simulink library "forceslib"  (R2020b)
settings: Solver=VariableStepAuto  StartTime=0.0  StopTime=10.0  RelTol=1e-3
undefined symbols (not defined in the file or in its folder): forcesnlmpcblock_InitFcn
settings Model: Creator=rchen  LastModifiedBy=NivethanYogarajah

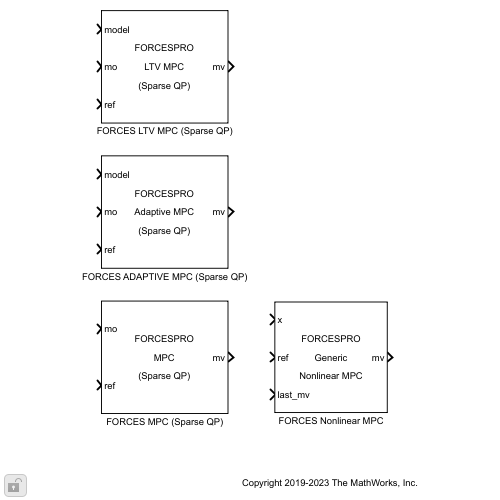
[thumbnail: Simulink's stored preview of the top-level diagram]
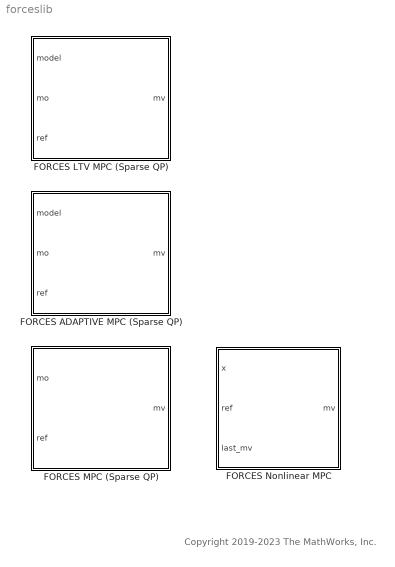
== system forceslib ==
  note: Copyright 2019-2023 The MathWorks, Inc.
  FORCES ADAPTIVE MPC (Sparse QP) : Subsystem  InitFcn=forcesmpcblock_InitFcn  mask(ForcesAdaptiveMPC_SparseQP){CoreData=[], StateData=[], md_inport=off, mv_inport=off, uref_inport=off, state_inport=off, ymin_inport=off, ymax_inport=off, umin_inport=off, umax_inport=off, dumin_inport=off, dumax_inport=off, ywt_inport=off, uwt_inport=off, duwt_inport=off, ecrwt_inport=off, return_cost=off, return_mvseq=off, return_qpstatus=off, return_qpsolvetime=off, return_solverid=off, return_xseq=off, return_state=off, return_yseq=off}
      mask prompts: CoreData "Core Data"; StateData "Initial State Data"; md_inport "Measured disturbance (md)"; mv_inport "External manipulated variable (ext.mv)"; uref_inport "References for manipulated variables (mv.target)"; state_inport "Use custom state estimation (x[k|k])"; ymin_inport "Lower OV Limits (ymin)"; ymax_inport "Upper OV Limits (ymax)"; umin_inport "Lower MV Limits (umin)"; umax_inport "Upper MV Limits (umax)"; dumin_inport "Lower MVRate Limits (dumin)"; dumax_inport "Upper MVRate Limits (dumax)"; ywt_inport "OV Weights (y.wt)"; uwt_inport "MV Weights (u.wt)"; duwt_inport "MVRate Weights (du.wt)"; ecrwt_inport "Slack Variable Weight (ecr.wt)"; return_cost "Optimal cost (cost)"; return_mvseq "Optimal control sequence (mv.seq)"; return_qpstatus "Optimization status (qp.status)"; return_qpsolvetime "Optimization solvetime (qp.solvetime)"; return_solverid "Solver Id (solverid)"; return_xseq "Optimal state sequence (x.seq)"; return_state "Estimated current states (est.state)"; return_yseq "Optimal output sequence (y.seq)"
      mask help:
      | Simulate adaptive MPC controller and generate code  using FORCESPRO QP solver.
      |
      | In MATLAB, use the following commands to generate custom FORCES QP solver from your MPC controller (mpcobj):
      |     options = mpcToForcesOptions('sparse');
      |     options.UseAdaptive = 1;
      |     [coredata, statedata, onlinedata] = mpcToForces(mpcobj, options);
      | You can enable additional online features via the "options".
      |
      | Afterwards, specify "coredata" and "statedata" in the block dialog and enable additional input and output signals in the block that must be consistent with "options".
      mask init:
      | BlockDataType = 'double';
      | MPCstruct = forcesmpcblock_MaskInitFcn(gcb);
      mask DialogControl Container5 Prompt: Additional Signal Configuration
      mask DialogControl Container7 Prompt: State Estimation
      mask DialogControl Container3 Prompt: Online Constraints
      mask DialogControl Container4 Prompt: Online Weights
      mask DialogControl Container9 Prompt: Additional Output Signals
      mask Display:
      | fprintf('FORCESPRO\n\nAdaptive MPC\n\n(Sparse QP)');
      | port_label('output', 1, 'mv')
      | port_label('input', 1, 'model')
      | port_label('input', 2, 'mo')
      | port_label('input', 3, 'ref')
  FORCES LTV MPC (Sparse QP) : Subsystem  InitFcn=forcesmpcblock_InitFcn  mask(ForcesLTVMPC_SparseQP){CoreData=[], StateData=[], md_inport=off, mv_inport=off, uref_inport=off, state_inport=off, ymin_inport=off, ymax_inport=off, umin_inport=off, umax_inport=off, dumin_inport=off, dumax_inport=off, ywt_inport=off, uwt_inport=off, duwt_inport=off, ecrwt_inport=off, return_cost=off, return_mvseq=off, return_qpstatus=off, return_qpsolvetime=off, return_solverid=off, return_xseq=off, return_state=off, return_yseq=off}
      mask prompts: CoreData "Core Data"; StateData "Initial State Data"; md_inport "Measured disturbance (md)"; mv_inport "External manipulated variable (ext.mv)"; uref_inport "References for manipulated variables (mv.target)"; state_inport "Use custom state estimation (x[k|k])"; ymin_inport "Lower OV Limits (ymin)"; ymax_inport "Upper OV Limits (ymax)"; umin_inport "Lower MV Limits (umin)"; umax_inport "Upper MV Limits (umax)"; dumin_inport "Lower MVRate Limits (dumin)"; dumax_inport "Upper MVRate Limits (dumax)"; ywt_inport "OV Weights (y.wt)"; uwt_inport "MV Weights (u.wt)"; duwt_inport "MVRate Weights (du.wt)"; ecrwt_inport "Slack Variable Weight (ecr.wt)"; return_cost "Optimal cost (cost)"; return_mvseq "Optimal control sequence (mv.seq)"; return_qpstatus "Optimization status (qp.status)"; return_qpsolvetime "Optimization solvetime (qp.solvetime)"; return_solverid "Solver Id (solverid)"; return_xseq "Optimal state sequence (x.seq)"; return_state "Estimated current states (est.state)"; return_yseq "Optimal output sequence (y.seq)"
      mask help:
      | Simulate time-varying MPC controller and generate code  using FORCESPRO QP solver.
      |
      | In MATLAB, use the following commands to generate custom FORCES QP solver from your MPC controller (mpcobj):
      |     options = mpcToForcesOptions('sparse');
      |     options.UseLTV = 1;
      |     [coredata, statedata, onlinedata] = mpcToForces(mpcobj, options);
      | You can enable additional online features via the "options".
      |
      | Afterwards, specify "coredata" and "statedata" in the block dialog and enable additional input and output signals in the block that must be consistent with "options".
      mask init:
      | BlockDataType = 'double';
      | MPCstruct = forcesmpcblock_MaskInitFcn(gcb);
      mask DialogControl Container5 Prompt: Additional Signal Configuration
      mask DialogControl Container7 Prompt: State Estimation
      mask DialogControl Container3 Prompt: Online Constraints
      mask DialogControl Container4 Prompt: Online Weights
      mask DialogControl Container9 Prompt: Additional Output Signals
      mask Display:
      | fprintf('FORCESPRO\n\nLTV MPC\n\n(Sparse QP)');
      | port_label('output', 1, 'mv')
      | port_label('input', 1, 'model')
      | port_label('input', 2, 'mo')
      | port_label('input', 3, 'ref')
  FORCES MPC (Sparse QP) : Subsystem  InitFcn=forcesmpcblock_InitFcn  mask(ForcesMPC_SparseQP){CoreData=[], StateData=[], md_inport=off, mv_inport=off, uref_inport=off, state_inport=off, ymin_inport=off, ymax_inport=off, umin_inport=off, umax_inport=off, dumin_inport=off, dumax_inport=off, ywt_inport=off, uwt_inport=off, duwt_inport=off, ecrwt_inport=off, return_cost=off, return_mvseq=off, return_qpstatus=off, return_qpsolvetime=off, return_solverid=off, return_xseq=off, return_state=off, return_yseq=off}
      mask prompts: CoreData "Core Data"; StateData "Initial State Data"; md_inport "Measured disturbance (md)"; mv_inport "External manipulated variable (ext.mv)"; uref_inport "References for manipulated variables (mv.target)"; state_inport "Use custom state estimation (x[k|k])"; ymin_inport "Lower OV Limits (ymin)"; ymax_inport "Upper OV Limits (ymax)"; umin_inport "Lower MV Limits (umin)"; umax_inport "Upper MV Limits (umax)"; dumin_inport "Lower MVRate Limits (dumin)"; dumax_inport "Upper MVRate Limits (dumax)"; ywt_inport "OV Weights (y.wt)"; uwt_inport "MV Weights (u.wt)"; duwt_inport "MVRate Weights (du.wt)"; ecrwt_inport "Slack Variable Weight (ecr.wt)"; return_cost "Optimal cost (cost)"; return_mvseq "Optimal control sequence (mv.seq)"; return_qpstatus "Optimization status (qp.status)"; return_qpsolvetime "Optimization solvetime (qp.solvetime)"; return_solverid "Solver Id (solverid)"; return_xseq "Optimal state sequence (x.seq)"; return_state "Estimated current states (est.state)"; return_yseq "Optimal output sequence (y.seq)"
      mask help:
      | Simulate MPC controller and generate code  using FORCESPRO QP solver.
      |
      | In MATLAB, use the following commands to generate custom FORCES QP solver from your MPC controller (mpcobj):
      |     options = mpcToForcesOptions('sparse');
      |     [coredata, statedata, onlinedata] = mpcToForces(mpcobj, options);
      | You can enable additional online features via the "options".
      |
      | Afterwards, specify "coredata" and "statedata" in the block dialog and enable additional input and output signals in the block that must be consistent with "options".
      mask init:
      | BlockDataType = 'double';
      | MPCstruct = forcesmpcblock_MaskInitFcn(gcb);
      mask DialogControl Container5 Prompt: Additional Signal Configuration
      mask DialogControl Container7 Prompt: State Estimation
      mask DialogControl Container3 Prompt: Online Constraints
      mask DialogControl Container4 Prompt: Online Weights
      mask DialogControl Container9 Prompt: Additional Output Signals
      mask Display:
      | fprintf('FORCESPRO\n\nMPC\n\n(Sparse QP)');
      | port_label('output', 1, 'mv')
      | port_label('input', 1, 'mo')
      | port_label('input', 2, 'ref')
  FORCES Nonlinear MPC : Subsystem  SCDEnableBlockLinearizationSpecification=on  InitFcn=forcesnlmpcblock_InitFcn;  mask(NonlinearMPC_FORCESPRO){nlmpcobj=, UseObjectTs=on, TsControl=, md_enabled=off, mvtarget_enabled=off, param_enabled=off, cost_enabled=off, mvseq_enabled=off, stateseq_enabled=off, ovseq_enabled=off, status_enabled=off, solvetime_enabled=off, solverid_enabled=off, ov_min=off, ov_max=off, mv_min=off, mv_max=off, mvrate_min=off, mvrate_max=off, state_min=off, state_max=off, ov_weight=off, mv_weight=off, mvrate_weight=off, ecr_weight=off, nlp_initialize=off}
      mask prompts: nlmpcobj ""coredata" structure generated from "nlmpcToForces""; UseObjectTs "Use prediction model sample time"; TsControl "Controller sample time (can be faster than prediction model sample time)"; md_enabled "Measured disturbances (md)"; mvtarget_enabled "MV targets (mv.target)"; param_enabled "Model parameters (param)"; cost_enabled "Optimal cost (cost)"; mvseq_enabled "Optimal control sequence (mv.seq)"; stateseq_enabled "Optimal state sequence (x.seq)"; ovseq_enabled "Optimal output sequence (y.seq)"; status_enabled "Optimization status (nlp.status)"; solvetime_enabled "Optimization solvetime (nlp.solvetime)"; solverid_enabled "Solver Id (solverid)"; ov_min "Lower OV limits (y.min)"; ov_max "Upper OV limits (y.max)"; mv_min "Lower MV limits (mv.min)"; mv_max "Upper MV limits (mv.max)"; mvrate_min "Lower MVRate limits (dmv.min)"; mvrate_max "Upper MVRate limits (dmv.max)"; state_min "Lower state limits (x.min)"; state_max "Upper state limits (x.max)"; ov_weight "OV weights (y.wt)"; mv_weight "MV weights (mv.wt)"; mvrate_weight "MVRate weights (dmv.wt)"; ecr_weight "ECR weight (ecr.wt)"; nlp_initialize "Initial guess (mv.init, x.init)"
      mask help:
      | Simulate nonlinear MPC controller designed with "nlmpc" object from MathWorks MPC Toolbox and generate code using FORCESPRO NLP solver.
      |
      | In MATLAB, use the following commands to generate FORCES NLP solver from your "nlmpc" controller (nlobj):
      |     options = nlmpcToForcesOptions();
      |     coredata = nlmpcToForces(nlobj, options);
      | You can enable additional online features via the "options".
      |
      | Afterwards, specify "coredata" in the block dialog and enable additional input and output signals in the block that must be consistent with "options".
      mask init:
      | BlockDataType = 'double';
      | blkData = forcesnlmpcblock_MaskInitFcn(gcb);
      mask Callback UseObjectTs: nlmpc.callbackBlockCustomSampleTime(gcb);
      mask DialogControl nlmpcobj Tooltip: Specify the "coredata" structure available in MATLAB workspace or Model workspace.
      mask DialogControl Container23 Prompt: Controller Sample Time
      mask DialogControl UseObjectTs Tooltip: Select if you want to run the Nonlinear MPC block using the same sample time as the prediction model sample time defined in the nlmpc object (a typical situation).
      mask DialogControl TsControl Tooltip: If you want to run the Nonlinear MPC block using sample time faster than the prediction model sample time defined in the nlmpc object, specify it here.
      mask DialogControl OptionGroup Prompt: Block Options
      mask DialogControl GeneralTab Prompt: General
      mask DialogControl Container6 Prompt: Additional Inports
      mask DialogControl md_enabled Tooltip: Select if the nlmpc object has measured disturbance (MD) channels. Connect MD signals to this input port.
      mask DialogControl mvtarget_enabled Tooltip: Select if you want to specify MV references at run time. Connect a [1..p]-by-nmv signal to the input port.
      mask DialogControl param_enabled Tooltip: Select if the nlmpc object has a model parameter and connect it with a vector signal
      mask DialogControl Container7 Prompt: Additional Outports
      mask DialogControl cost_enabled Tooltip: Select if you want to access the optimal cost as a scalar signal.
      mask DialogControl mvseq_enabled Tooltip: Select if you want to access the optimal control move trajectory as a (p+1)-by-nmv signal.
      mask DialogControl stateseq_enabled Tooltip: Select if you want to access the predicted state trajectory as a (p+1)-by-nx signal.
      mask DialogControl ovseq_enabled Tooltip: Select if you want to access the predicted output trajectory as a (p+1)-by-ny signal.
      mask DialogControl status_enabled Tooltip: Select if you want to access the optimization status as a scalar signal. A positive integer indicates the solver found an optimal solution. A negative integer indicates the solver failed to find a solution, and the mv output was frozen. Zero value indicates that the maximum number of iterations was exceeded.
      mask DialogControl solvetime_enabled Tooltip: Select if you want to access the optimization status as a scalar signal. A positive integer indicates the solver found an optimal solution. A negative integer indicates the solver failed to find a solution, and the mv output was frozen. Zero value indicates that the maximum number of iterations was exceeded.
      mask DialogControl solverid_enabled Tooltip: Select if you want to access the optimization status as a scalar signal. A positive integer indicates the solver found an optimal solution. A negative integer indicates the solver failed to find a solution, and the mv output was frozen. Zero value indicates that the maximum number of iterations was exceeded.
      mask DialogControl OnlineTab Prompt: Online Features
      mask DialogControl Container6_copy Prompt: Constraints
      mask DialogControl ov_min Tooltip: Select if you want to change the minimum OV bound at run time. Connect a [1..p]-by-ny signal to the input port.
      mask DialogControl ov_max Tooltip: Select if you want to change the maximum OV bound at run time. Connect a [1..p]-by-ny signal to the input port.
      mask DialogControl mv_min Tooltip: Select if you want to change the minimum MV bound at run time. Connect a [1..p]-by-nmv signal to the input port.
      mask DialogControl mv_max Tooltip: Select if you want to change the maximum MV bound at run time. Connect a [1..p]-by-nmv signal to the input port.
      mask DialogControl mvrate_min Tooltip: Select if you want to change the minimum MVRate bound at run time. Connect a [1..p]-by-nmv signal to the input port.
      mask DialogControl mvrate_max Tooltip: Select if you want to change the maximum MVRate bound at run time. Connect a [1..p]-by-nmv signal to the input port.
      mask DialogControl state_min Tooltip: Select if you want to change the minimum state bound at run time. Connect a [1..p]-by-nx signal to the input port.
      mask DialogControl state_max Tooltip: Select if you want to change the maximum state bound at run time. Connect a [1..p]-by-nx signal to the input port.
      mask DialogControl Container7_copy Prompt: Weights
      mask DialogControl ov_weight Tooltip: Select if you want to change OV weights at run time. Connect a (1..p)-by-ny signal to the input port.
      mask DialogControl mv_weight Tooltip: Select if you want to change MV weights at run time. Connect a (1..p)-by-nmv signal to the input port.
      mask DialogControl mvrate_weight Tooltip: Select if you want to change MVRate weights at run time. Connect a (1..p)-by-nmv signal to the input port.
      mask DialogControl ecr_weight Tooltip: Select if you want to change ECR weight at run time. Connect a scalar signal to the input port.
      mask DialogControl Container13 Prompt: Others
      mask DialogControl nlp_initialize Tooltip: Select if you want to provide your own initial guess for the decision variables used in optimization at run time. Connect a "p-by-nx" signal to "x.init" and a "p-by-nmv" signal to "mv.init".
      mask Display:
      | fprintf('FORCESPRO\n\nGeneric\n\nNonlinear MPC');
      | port_label('output', 1, 'mv')
      | port_label('input', 1, 'x')
      | port_label('input', 2, 'ref')
      | port_label('input', 3, 'last_mv')

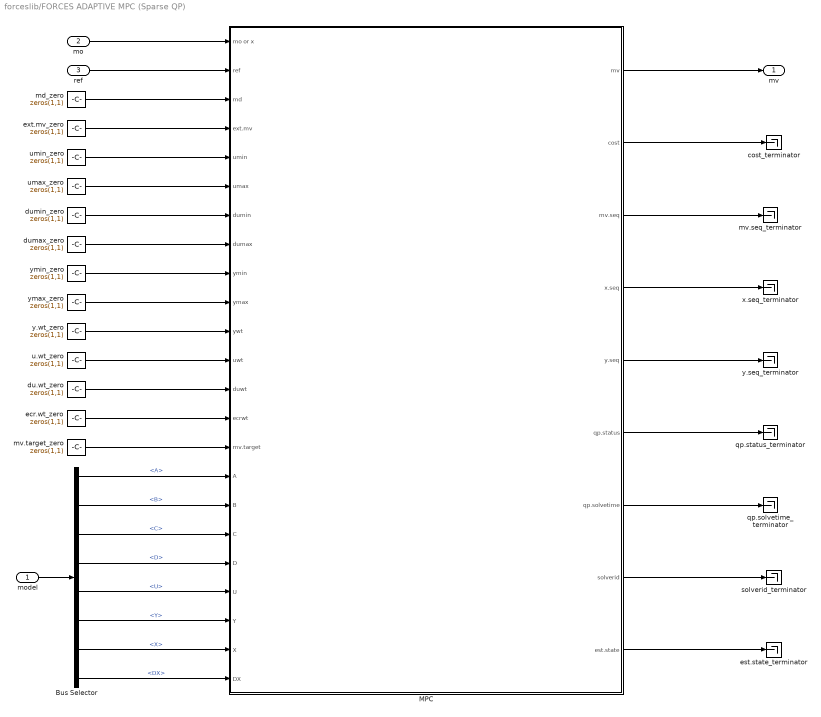
== system forceslib/FORCES ADAPTIVE MPC (Sparse QP) ==
  model : Inport
  mo : Inport  Port=2
  ref : Inport  Port=3
  Bus Selector : BusSelector  OutputSignals=A,B,C,D,U,Y,X,DX
  MPC : Subsystem
  cost_terminator : Terminator
  du.wt_zero : Constant  Value=zeros(1,1)  OutDataTypeStr=BlockDataType  SampleTime=-1
  dumax_zero : Constant  Value=zeros(1,1)  OutDataTypeStr=BlockDataType  SampleTime=-1
  dumin_zero : Constant  Value=zeros(1,1)  OutDataTypeStr=BlockDataType  SampleTime=-1
  ecr.wt_zero : Constant  Value=zeros(1,1)  OutDataTypeStr=BlockDataType  SampleTime=-1
  est.state_terminator : Terminator
  ext.mv_zero : Constant  Value=zeros(1,1)  OutDataTypeStr=BlockDataType  SampleTime=-1
  md_zero : Constant  Value=zeros(1,1)  OutDataTypeStr=BlockDataType  SampleTime=-1
  mv.seq_terminator : Terminator
  mv.target_zero : Constant  Value=zeros(1,1)  OutDataTypeStr=BlockDataType  SampleTime=-1
  qp.solvetime_terminator : Terminator
  qp.status_terminator : Terminator
  solverid_terminator : Terminator
  u.wt_zero : Constant  Value=zeros(1,1)  OutDataTypeStr=BlockDataType  SampleTime=-1
  umax_zero : Constant  Value=zeros(1,1)  OutDataTypeStr=BlockDataType  SampleTime=-1
  umin_zero : Constant  Value=zeros(1,1)  OutDataTypeStr=BlockDataType  SampleTime=-1
  x.seq_terminator : Terminator
  y.seq_terminator : Terminator
  y.wt_zero : Constant  Value=zeros(1,1)  OutDataTypeStr=BlockDataType  SampleTime=-1
  ymax_zero : Constant  Value=zeros(1,1)  OutDataTypeStr=BlockDataType  SampleTime=-1
  ymin_zero : Constant  Value=zeros(1,1)  OutDataTypeStr=BlockDataType  SampleTime=-1
  mv : Outport
  wires:
  MPC/7(qp.solvetime) -> qp.solvetime_terminator/1
  MPC/6(qp.status) -> qp.status_terminator/1
  MPC/5(y.seq) -> y.seq_terminator/1
  MPC/4(x.seq) -> x.seq_terminator/1
  MPC/3(mv.seq) -> mv.seq_terminator/1
  MPC/2(cost) -> cost_terminator/1
  mv.target_zero/1 -> MPC/15(mv.target)
  ecr.wt_zero/1 -> MPC/14(ecrwt)
  du.wt_zero/1 -> MPC/13(duwt)
  u.wt_zero/1 -> MPC/12(uwt)
  y.wt_zero/1 -> MPC/11(ywt)
  ymax_zero/1 -> MPC/10(ymax)
  ymin_zero/1 -> MPC/9(ymin)
  dumax_zero/1 -> MPC/8(dumax)
  dumin_zero/1 -> MPC/7(dumin)
  umax_zero/1 -> MPC/6(umax)
  umin_zero/1 -> MPC/5(umin)
  ext.mv_zero/1 -> MPC/4(ext.mv)
  md_zero/1 -> MPC/3(md)
  MPC/1(mv) -> mv/1
  ref/1 -> MPC/2(ref)
  mo/1 -> MPC/1(mo or x)
  MPC/9(est.state) -> est.state_terminator/1
  MPC/8(solverid) -> solverid_terminator/1
  model/1 -> Bus Selector/1
  Bus Selector/1 -> MPC/16(A)  "<A>"
  Bus Selector/2 -> MPC/17(B)  "<B>"
  Bus Selector/3 -> MPC/18(C)  "<C>"
  Bus Selector/4 -> MPC/19(D)  "<D>"
  Bus Selector/5 -> MPC/20(U)  "<U>"
  Bus Selector/6 -> MPC/21(Y)  "<Y>"
  Bus Selector/7 -> MPC/22(X)  "<X>"
  Bus Selector/8 -> MPC/23(DX)  "<DX>"

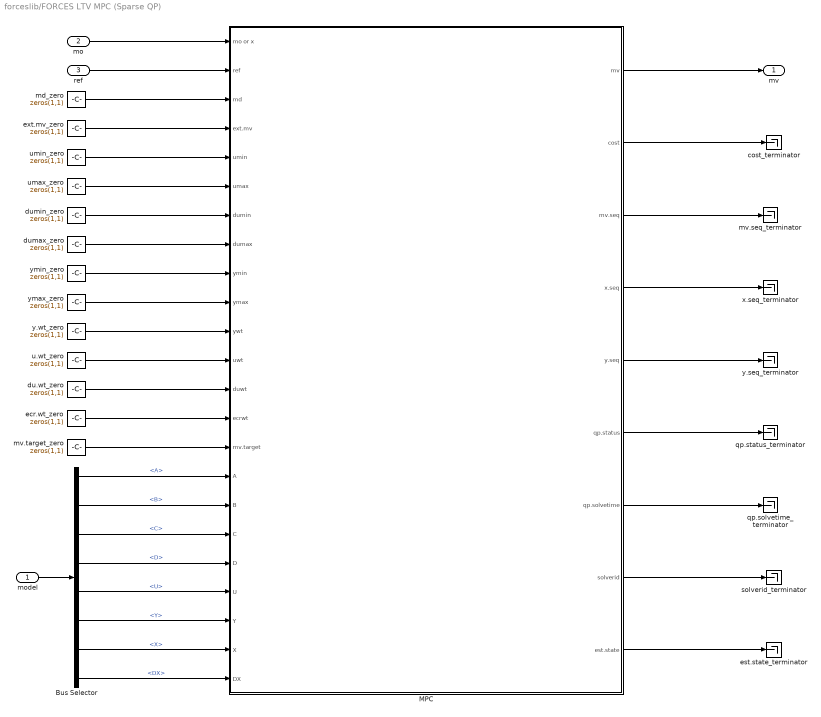
== system forceslib/FORCES LTV MPC (Sparse QP) ==
  model : Inport
  mo : Inport  Port=2
  ref : Inport  Port=3
  Bus Selector : BusSelector  OutputSignals=A,B,C,D,U,Y,X,DX
  MPC : Subsystem
  cost_terminator : Terminator
  du.wt_zero : Constant  Value=zeros(1,1)  OutDataTypeStr=BlockDataType  SampleTime=-1
  dumax_zero : Constant  Value=zeros(1,1)  OutDataTypeStr=BlockDataType  SampleTime=-1
  dumin_zero : Constant  Value=zeros(1,1)  OutDataTypeStr=BlockDataType  SampleTime=-1
  ecr.wt_zero : Constant  Value=zeros(1,1)  OutDataTypeStr=BlockDataType  SampleTime=-1
  est.state_terminator : Terminator
  ext.mv_zero : Constant  Value=zeros(1,1)  OutDataTypeStr=BlockDataType  SampleTime=-1
  md_zero : Constant  Value=zeros(1,1)  OutDataTypeStr=BlockDataType  SampleTime=-1
  mv.seq_terminator : Terminator
  mv.target_zero : Constant  Value=zeros(1,1)  OutDataTypeStr=BlockDataType  SampleTime=-1
  qp.solvetime_terminator : Terminator
  qp.status_terminator : Terminator
  solverid_terminator : Terminator
  u.wt_zero : Constant  Value=zeros(1,1)  OutDataTypeStr=BlockDataType  SampleTime=-1
  umax_zero : Constant  Value=zeros(1,1)  OutDataTypeStr=BlockDataType  SampleTime=-1
  umin_zero : Constant  Value=zeros(1,1)  OutDataTypeStr=BlockDataType  SampleTime=-1
  x.seq_terminator : Terminator
  y.seq_terminator : Terminator
  y.wt_zero : Constant  Value=zeros(1,1)  OutDataTypeStr=BlockDataType  SampleTime=-1
  ymax_zero : Constant  Value=zeros(1,1)  OutDataTypeStr=BlockDataType  SampleTime=-1
  ymin_zero : Constant  Value=zeros(1,1)  OutDataTypeStr=BlockDataType  SampleTime=-1
  mv : Outport
  wires:
  MPC/7(qp.solvetime) -> qp.solvetime_terminator/1
  MPC/6(qp.status) -> qp.status_terminator/1
  MPC/5(y.seq) -> y.seq_terminator/1
  MPC/4(x.seq) -> x.seq_terminator/1
  MPC/3(mv.seq) -> mv.seq_terminator/1
  MPC/2(cost) -> cost_terminator/1
  mv.target_zero/1 -> MPC/15(mv.target)
  ecr.wt_zero/1 -> MPC/14(ecrwt)
  du.wt_zero/1 -> MPC/13(duwt)
  u.wt_zero/1 -> MPC/12(uwt)
  y.wt_zero/1 -> MPC/11(ywt)
  ymax_zero/1 -> MPC/10(ymax)
  ymin_zero/1 -> MPC/9(ymin)
  dumax_zero/1 -> MPC/8(dumax)
  dumin_zero/1 -> MPC/7(dumin)
  umax_zero/1 -> MPC/6(umax)
  umin_zero/1 -> MPC/5(umin)
  ext.mv_zero/1 -> MPC/4(ext.mv)
  md_zero/1 -> MPC/3(md)
  MPC/1(mv) -> mv/1
  ref/1 -> MPC/2(ref)
  mo/1 -> MPC/1(mo or x)
  MPC/9(est.state) -> est.state_terminator/1
  MPC/8(solverid) -> solverid_terminator/1
  model/1 -> Bus Selector/1
  Bus Selector/1 -> MPC/16(A)  "<A>"
  Bus Selector/2 -> MPC/17(B)  "<B>"
  Bus Selector/3 -> MPC/18(C)  "<C>"
  Bus Selector/4 -> MPC/19(D)  "<D>"
  Bus Selector/5 -> MPC/20(U)  "<U>"
  Bus Selector/6 -> MPC/21(Y)  "<Y>"
  Bus Selector/7 -> MPC/22(X)  "<X>"
  Bus Selector/8 -> MPC/23(DX)  "<DX>"

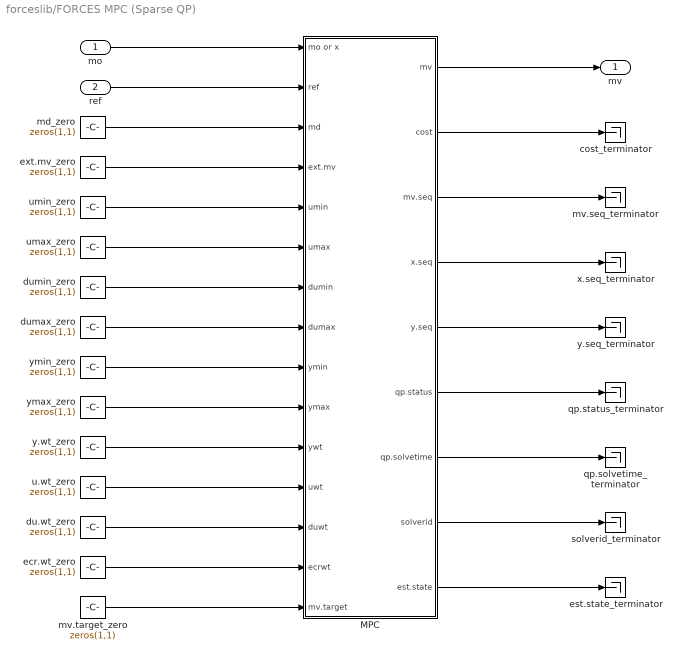
== system forceslib/FORCES MPC (Sparse QP) ==
  mo : Inport
  ref : Inport  Port=2
  MPC : Subsystem
  cost_terminator : Terminator
  du.wt_zero : Constant  Value=zeros(1,1)  OutDataTypeStr=BlockDataType  SampleTime=-1
  dumax_zero : Constant  Value=zeros(1,1)  OutDataTypeStr=BlockDataType  SampleTime=-1
  dumin_zero : Constant  Value=zeros(1,1)  OutDataTypeStr=BlockDataType  SampleTime=-1
  ecr.wt_zero : Constant  Value=zeros(1,1)  OutDataTypeStr=BlockDataType  SampleTime=-1
  est.state_terminator : Terminator
  ext.mv_zero : Constant  Value=zeros(1,1)  OutDataTypeStr=BlockDataType  SampleTime=-1
  md_zero : Constant  Value=zeros(1,1)  OutDataTypeStr=BlockDataType  SampleTime=-1
  mv.seq_terminator : Terminator
  mv.target_zero : Constant  Value=zeros(1,1)  OutDataTypeStr=BlockDataType  SampleTime=-1
  qp.solvetime_terminator : Terminator
  qp.status_terminator : Terminator
  solverid_terminator : Terminator
  u.wt_zero : Constant  Value=zeros(1,1)  OutDataTypeStr=BlockDataType  SampleTime=-1
  umax_zero : Constant  Value=zeros(1,1)  OutDataTypeStr=BlockDataType  SampleTime=-1
  umin_zero : Constant  Value=zeros(1,1)  OutDataTypeStr=BlockDataType  SampleTime=-1
  x.seq_terminator : Terminator
  y.seq_terminator : Terminator
  y.wt_zero : Constant  Value=zeros(1,1)  OutDataTypeStr=BlockDataType  SampleTime=-1
  ymax_zero : Constant  Value=zeros(1,1)  OutDataTypeStr=BlockDataType  SampleTime=-1
  ymin_zero : Constant  Value=zeros(1,1)  OutDataTypeStr=BlockDataType  SampleTime=-1
  mv : Outport
  wires:
  MPC/7(qp.solvetime) -> qp.solvetime_terminator/1
  MPC/6(qp.status) -> qp.status_terminator/1
  MPC/5(y.seq) -> y.seq_terminator/1
  MPC/4(x.seq) -> x.seq_terminator/1
  MPC/3(mv.seq) -> mv.seq_terminator/1
  MPC/2(cost) -> cost_terminator/1
  mv.target_zero/1 -> MPC/15(mv.target)
  ecr.wt_zero/1 -> MPC/14(ecrwt)
  du.wt_zero/1 -> MPC/13(duwt)
  u.wt_zero/1 -> MPC/12(uwt)
  y.wt_zero/1 -> MPC/11(ywt)
  ymax_zero/1 -> MPC/10(ymax)
  ymin_zero/1 -> MPC/9(ymin)
  dumax_zero/1 -> MPC/8(dumax)
  dumin_zero/1 -> MPC/7(dumin)
  umax_zero/1 -> MPC/6(umax)
  umin_zero/1 -> MPC/5(umin)
  ext.mv_zero/1 -> MPC/4(ext.mv)
  md_zero/1 -> MPC/3(md)
  MPC/1(mv) -> mv/1
  ref/1 -> MPC/2(ref)
  mo/1 -> MPC/1(mo or x)
  MPC/9(est.state) -> est.state_terminator/1
  MPC/8(solverid) -> solverid_terminator/1

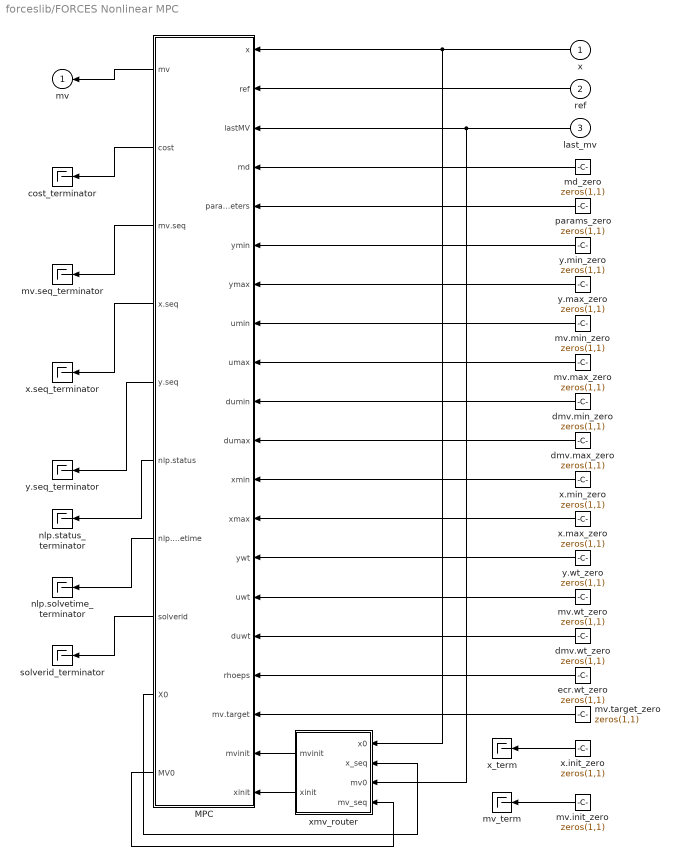
== system forceslib/FORCES Nonlinear MPC ==
  x : Inport
  ref : Inport  Port=2
  last_mv : Inport  Port=3
  MPC : Subsystem
  cost_terminator : Terminator
  dmv.max_zero : Constant  Value=zeros(1,1)
  dmv.min_zero : Constant  Value=zeros(1,1)
  dmv.wt_zero : Constant  Value=zeros(1,1)
  ecr.wt_zero : Constant  Value=zeros(1,1)
  md_zero : Constant  Value=zeros(1,1)  OutDataTypeStr=BlockDataType
  mv.init_zero : Constant  Value=zeros(1,1)  OutDataTypeStr=BlockDataType
  mv.max_zero : Constant  Value=zeros(1,1)
  mv.min_zero : Constant  Value=zeros(1,1)
  mv.seq_terminator : Terminator
  mv.target_zero : Constant  Value=zeros(1,1)  OutDataTypeStr=BlockDataType
  mv.wt_zero : Constant  Value=zeros(1,1)
  mv_term : Terminator
  nlp.solvetime_terminator : Terminator
  nlp.status_terminator : Terminator
  params_zero : Constant  Value=zeros(1,1)  OutDataTypeStr=BlockDataType
  solverid_terminator : Terminator
  x.init_zero : Constant  Value=zeros(1,1)  OutDataTypeStr=BlockDataType
  x.max_zero : Constant  Value=zeros(1,1)
  x.min_zero : Constant  Value=zeros(1,1)
  x.seq_terminator : Terminator
  x_term : Terminator
  xmv_router : Subsystem  mask{PredictionHorizon=blkData.p, Ts=blkData.Ts}
      mask prompts: PredictionHorizon "Prediction horizon"; Ts "Sample time"
  y.max_zero : Constant  Value=zeros(1,1)
  y.min_zero : Constant  Value=zeros(1,1)
  y.seq_terminator : Terminator
  y.wt_zero : Constant  Value=zeros(1,1)
  mv : Outport  VectorParamsAs1DForOutWhenUnconnected=off
  wires:
  mv.target_zero/1 -> MPC/18(mv.target)
  params_zero/1 -> MPC/5(parameters)
  md_zero/1 -> MPC/4(md)
  mv.init_zero/1 -> mv_term/1
  x.init_zero/1 -> x_term/1
  MPC/10(MV0) -> xmv_router/4(mv_seq)
  MPC/9(X0) -> xmv_router/2(x_seq)
  xmv_router/2(xinit) -> MPC/20(xinit)
  xmv_router/1(mvinit) -> MPC/19(mvinit)
  ref/1 -> MPC/2(ref)
  x/1 -> MPC/1(x), xmv_router/1(x0)
  MPC/1(mv) -> mv/1
  last_mv/1 -> MPC/3(lastMV), xmv_router/3(mv0)
  MPC/2(cost) -> cost_terminator/1
  MPC/3(mv.seq) -> mv.seq_terminator/1
  MPC/4(x.seq) -> x.seq_terminator/1
  MPC/5(y.seq) -> y.seq_terminator/1
  mv.min_zero/1 -> MPC/8(umin)
  mv.max_zero/1 -> MPC/9(umax)
  y.min_zero/1 -> MPC/6(ymin)
  y.max_zero/1 -> MPC/7(ymax)
  x.min_zero/1 -> MPC/12(xmin)
  x.max_zero/1 -> MPC/13(xmax)
  y.wt_zero/1 -> MPC/14(ywt)
  mv.wt_zero/1 -> MPC/15(uwt)
  dmv.wt_zero/1 -> MPC/16(duwt)
  MPC/6(nlp.status) -> nlp.status_terminator/1
  dmv.min_zero/1 -> MPC/10(dumin)
  dmv.max_zero/1 -> MPC/11(dumax)
  ecr.wt_zero/1 -> MPC/17(rhoeps)
  MPC/7(nlp.solvetime) -> nlp.solvetime_terminator/1
  MPC/8(solverid) -> solverid_terminator/1

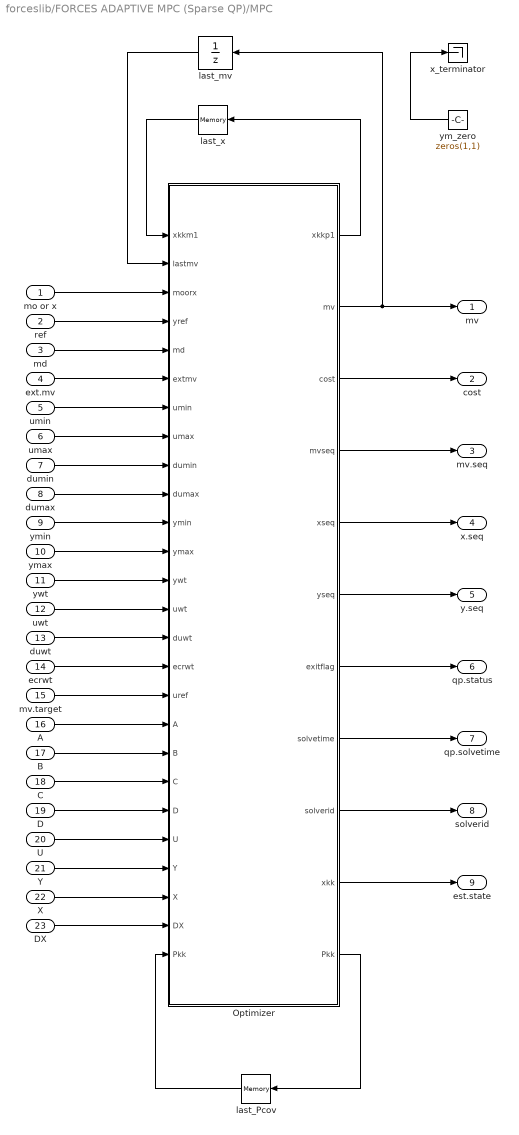
== system forceslib/FORCES ADAPTIVE MPC (Sparse QP)/MPC ==
  mo or x : Inport
  ref : Inport  Port=2
  md : Inport  Port=3
  ext.mv : Inport  Port=4
  umin : Inport  Port=5
  umax : Inport  Port=6
  dumin : Inport  Port=7
  dumax : Inport  Port=8
  ymin : Inport  Port=9
  ymax : Inport  Port=10
  ywt : Inport  Port=11
  uwt : Inport  Port=12
  duwt : Inport  Port=13
  ecrwt : Inport  Port=14
  mv.target : Inport  Port=15
  A : Inport  Port=16
  B : Inport  Port=17
  C : Inport  Port=18
  D : Inport  Port=19
  U : Inport  Port=20
  Y : Inport  Port=21
  X : Inport  Port=22
  DX : Inport  Port=23
  Optimizer : MATLAB Function  TreatAsAtomicUnit=on
  last_Pcov : Memory  InitialCondition=MPCstruct.P0  InheritSampleTime=on  LinearizeAsDelay=on
  last_mv : UnitDelay  InitialCondition=MPCstruct.MV0  SampleTime=-1  HasFrameUpgradeWarning=on
  last_x : Memory  InitialCondition=MPCstruct.X0  InheritSampleTime=on  LinearizeAsDelay=on
  x_terminator : Terminator
  ym_zero : Constant  Value=zeros(1,1)  OutDataTypeStr=BlockDataType
  mv : Outport
  cost : Outport  Port=2
  mv.seq : Outport  Port=3
  x.seq : Outport  Port=4
  y.seq : Outport  Port=5
  qp.status : Outport  Port=6
  qp.solvetime : Outport  Port=7
  solverid : Outport  Port=8
  est.state : Outport  Port=9
  wires:
  ref/1 -> Optimizer/4(yref)
  Optimizer/3(cost) -> cost/1
  Optimizer/4(mvseq) -> mv.seq/1
  Optimizer/5(xseq) -> x.seq/1
  Optimizer/6(yseq) -> y.seq/1
  Optimizer/7(exitflag) -> qp.status/1
  Optimizer/10(xkk) -> est.state/1
  ymax/1 -> Optimizer/12(ymax)
  ymin/1 -> Optimizer/11(ymin)
  dumax/1 -> Optimizer/10(dumax)
  dumin/1 -> Optimizer/9(dumin)
  umax/1 -> Optimizer/8(umax)
  umin/1 -> Optimizer/7(umin)
  ext.mv/1 -> Optimizer/6(extmv)
  md/1 -> Optimizer/5(md)
  duwt/1 -> Optimizer/15(duwt)
  uwt/1 -> Optimizer/14(uwt)
  ywt/1 -> Optimizer/13(ywt)
  ecrwt/1 -> Optimizer/16(ecrwt)
  mv.target/1 -> Optimizer/17(uref)
  ym_zero/1 -> x_terminator/1
  last_mv/1 -> Optimizer/2(lastmv)
  Optimizer/1(xkkp1) -> last_x/1
  last_x/1 -> Optimizer/1(xkkm1)
  Optimizer/2(mv) -> mv/1, last_mv/1
  mo or x/1 -> Optimizer/3(moorx)
  Optimizer/8(solvetime) -> qp.solvetime/1
  Optimizer/9(solverid) -> solverid/1
  last_Pcov/1 -> Optimizer/26("Pkk ")
  DX/1 -> Optimizer/25(DX)
  B/1 -> Optimizer/19(B)
  C/1 -> Optimizer/20(C)
  Y/1 -> Optimizer/23(Y)
  D/1 -> Optimizer/21(D)
  A/1 -> Optimizer/18(A)
  U/1 -> Optimizer/22(U)
  X/1 -> Optimizer/24(X)
  Optimizer/11(Pkk) -> last_Pcov/1

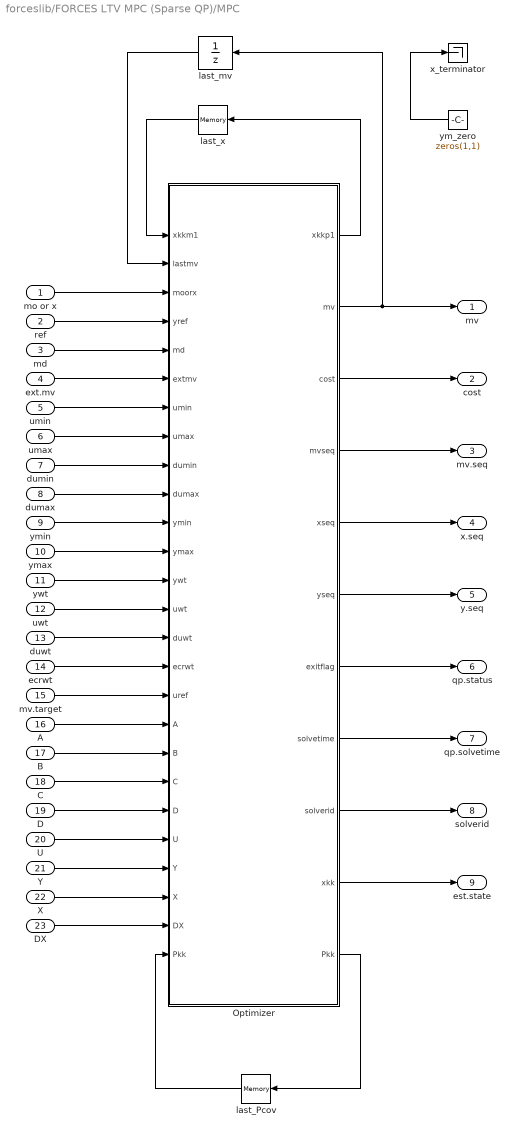
== system forceslib/FORCES LTV MPC (Sparse QP)/MPC ==
  mo or x : Inport
  ref : Inport  Port=2
  md : Inport  Port=3
  ext.mv : Inport  Port=4
  umin : Inport  Port=5
  umax : Inport  Port=6
  dumin : Inport  Port=7
  dumax : Inport  Port=8
  ymin : Inport  Port=9
  ymax : Inport  Port=10
  ywt : Inport  Port=11
  uwt : Inport  Port=12
  duwt : Inport  Port=13
  ecrwt : Inport  Port=14
  mv.target : Inport  Port=15
  A : Inport  Port=16
  B : Inport  Port=17
  C : Inport  Port=18
  D : Inport  Port=19
  U : Inport  Port=20
  Y : Inport  Port=21
  X : Inport  Port=22
  DX : Inport  Port=23
  Optimizer : MATLAB Function  TreatAsAtomicUnit=on
  last_Pcov : Memory  InitialCondition=MPCstruct.P0  InheritSampleTime=on  LinearizeAsDelay=on
  last_mv : UnitDelay  InitialCondition=MPCstruct.MV0  SampleTime=-1  HasFrameUpgradeWarning=on
  last_x : Memory  InitialCondition=MPCstruct.X0  InheritSampleTime=on  LinearizeAsDelay=on
  x_terminator : Terminator
  ym_zero : Constant  Value=zeros(1,1)  OutDataTypeStr=BlockDataType
  mv : Outport
  cost : Outport  Port=2
  mv.seq : Outport  Port=3
  x.seq : Outport  Port=4
  y.seq : Outport  Port=5
  qp.status : Outport  Port=6
  qp.solvetime : Outport  Port=7
  solverid : Outport  Port=8
  est.state : Outport  Port=9
  wires:
  ref/1 -> Optimizer/4(yref)
  Optimizer/3(cost) -> cost/1
  Optimizer/4(mvseq) -> mv.seq/1
  Optimizer/5(xseq) -> x.seq/1
  Optimizer/6(yseq) -> y.seq/1
  Optimizer/7(exitflag) -> qp.status/1
  Optimizer/10(xkk) -> est.state/1
  ymax/1 -> Optimizer/12(ymax)
  ymin/1 -> Optimizer/11(ymin)
  dumax/1 -> Optimizer/10(dumax)
  dumin/1 -> Optimizer/9(dumin)
  umax/1 -> Optimizer/8(umax)
  umin/1 -> Optimizer/7(umin)
  ext.mv/1 -> Optimizer/6(extmv)
  md/1 -> Optimizer/5(md)
  duwt/1 -> Optimizer/15(duwt)
  uwt/1 -> Optimizer/14(uwt)
  ywt/1 -> Optimizer/13(ywt)
  ecrwt/1 -> Optimizer/16(ecrwt)
  mv.target/1 -> Optimizer/17(uref)
  ym_zero/1 -> x_terminator/1
  last_mv/1 -> Optimizer/2(lastmv)
  Optimizer/1(xkkp1) -> last_x/1
  last_x/1 -> Optimizer/1(xkkm1)
  Optimizer/2(mv) -> mv/1, last_mv/1
  mo or x/1 -> Optimizer/3(moorx)
  Optimizer/8(solvetime) -> qp.solvetime/1
  Optimizer/9(solverid) -> solverid/1
  last_Pcov/1 -> Optimizer/26("Pkk ")
  DX/1 -> Optimizer/25(DX)
  B/1 -> Optimizer/19(B)
  C/1 -> Optimizer/20(C)
  Y/1 -> Optimizer/23(Y)
  D/1 -> Optimizer/21(D)
  A/1 -> Optimizer/18(A)
  U/1 -> Optimizer/22(U)
  X/1 -> Optimizer/24(X)
  Optimizer/11(Pkk) -> last_Pcov/1

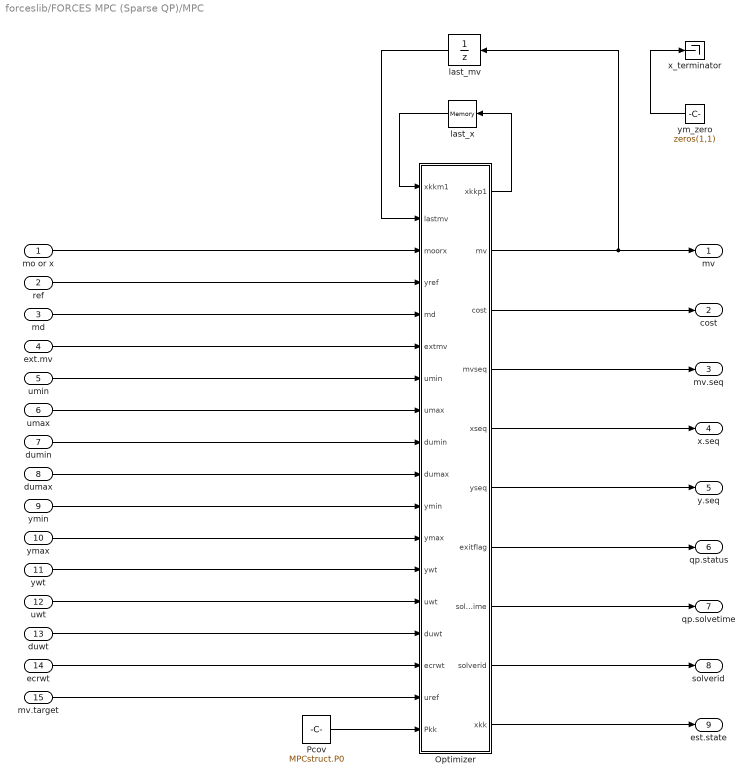
== system forceslib/FORCES MPC (Sparse QP)/MPC ==
  mo or x : Inport
  ref : Inport  Port=2
  md : Inport  Port=3
  ext.mv : Inport  Port=4
  umin : Inport  Port=5
  umax : Inport  Port=6
  dumin : Inport  Port=7
  dumax : Inport  Port=8
  ymin : Inport  Port=9
  ymax : Inport  Port=10
  ywt : Inport  Port=11
  uwt : Inport  Port=12
  duwt : Inport  Port=13
  ecrwt : Inport  Port=14
  mv.target : Inport  Port=15
  Optimizer : MATLAB Function  TreatAsAtomicUnit=on
  Pcov : Constant  Value=MPCstruct.P0
  last_mv : UnitDelay  InitialCondition=MPCstruct.MV0  SampleTime=-1  HasFrameUpgradeWarning=on
  last_x : Memory  InitialCondition=MPCstruct.X0  InheritSampleTime=on  LinearizeAsDelay=on
  x_terminator : Terminator
  ym_zero : Constant  Value=zeros(1,1)  OutDataTypeStr=BlockDataType
  mv : Outport
  cost : Outport  Port=2
  mv.seq : Outport  Port=3
  x.seq : Outport  Port=4
  y.seq : Outport  Port=5
  qp.status : Outport  Port=6
  qp.solvetime : Outport  Port=7
  solverid : Outport  Port=8
  est.state : Outport  Port=9
  wires:
  ref/1 -> Optimizer/4(yref)
  Optimizer/3(cost) -> cost/1
  Optimizer/4(mvseq) -> mv.seq/1
  Optimizer/5(xseq) -> x.seq/1
  Optimizer/6(yseq) -> y.seq/1
  Optimizer/7(exitflag) -> qp.status/1
  Optimizer/10(xkk) -> est.state/1
  ymax/1 -> Optimizer/12(ymax)
  ymin/1 -> Optimizer/11(ymin)
  dumax/1 -> Optimizer/10(dumax)
  dumin/1 -> Optimizer/9(dumin)
  umax/1 -> Optimizer/8(umax)
  umin/1 -> Optimizer/7(umin)
  ext.mv/1 -> Optimizer/6(extmv)
  md/1 -> Optimizer/5(md)
  duwt/1 -> Optimizer/15(duwt)
  uwt/1 -> Optimizer/14(uwt)
  ywt/1 -> Optimizer/13(ywt)
  ecrwt/1 -> Optimizer/16(ecrwt)
  mv.target/1 -> Optimizer/17(uref)
  ym_zero/1 -> x_terminator/1
  last_mv/1 -> Optimizer/2(lastmv)
  Optimizer/1(xkkp1) -> last_x/1
  last_x/1 -> Optimizer/1(xkkm1)
  Optimizer/2(mv) -> mv/1, last_mv/1
  mo or x/1 -> Optimizer/3(moorx)
  Optimizer/8(solvetime) -> qp.solvetime/1
  Optimizer/9(solverid) -> solverid/1
  Pcov/1 -> Optimizer/18(Pkk)

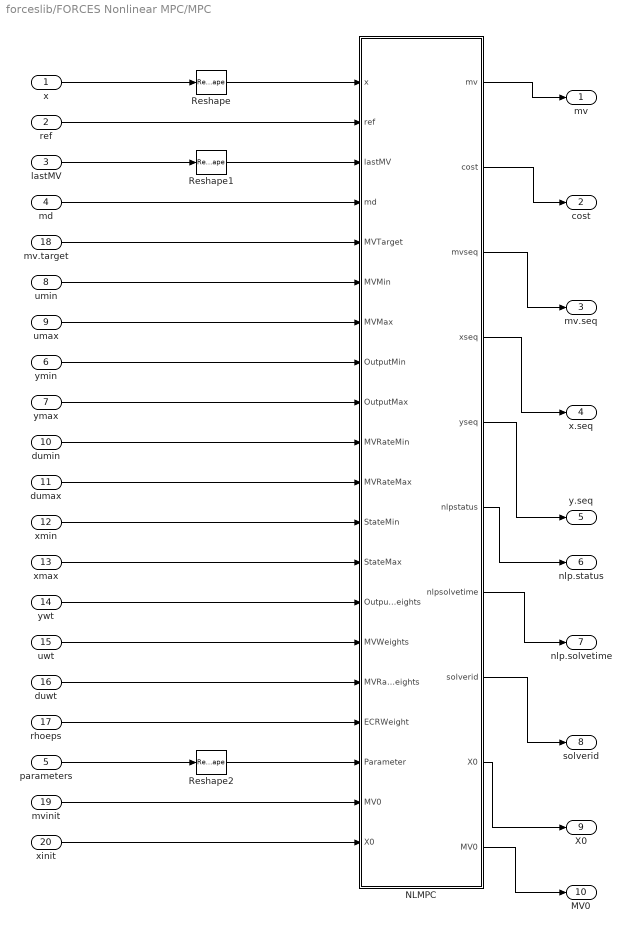
== system forceslib/FORCES Nonlinear MPC/MPC ==
  x : Inport
  ref : Inport  Port=2
  lastMV : Inport  Port=3
  md : Inport  Port=4
  parameters : Inport  Port=5
  ymin : Inport  Port=6
  ymax : Inport  Port=7
  umin : Inport  Port=8
  umax : Inport  Port=9
  dumin : Inport  Port=10
  dumax : Inport  Port=11
  xmin : Inport  Port=12
  xmax : Inport  Port=13
  ywt : Inport  Port=14
  uwt : Inport  Port=15
  duwt : Inport  Port=16
  rhoeps : Inport  Port=17
  mv.target : Inport  Port=18
  mvinit : Inport  Port=19
  xinit : Inport  Port=20
  NLMPC : MATLAB Function  TreatAsAtomicUnit=on
  Reshape : Reshape  OutputDimensionality=Column vector (2-D)
  Reshape1 : Reshape  OutputDimensionality=Column vector (2-D)
  Reshape2 : Reshape  OutputDimensionality=Column vector (2-D)
  mv : Outport  VectorParamsAs1DForOutWhenUnconnected=off
  cost : Outport  Port=2  VectorParamsAs1DForOutWhenUnconnected=off
  mv.seq : Outport  Port=3  VectorParamsAs1DForOutWhenUnconnected=off
  x.seq : Outport  Port=4  VectorParamsAs1DForOutWhenUnconnected=off
  y.seq : Outport  Port=5  VectorParamsAs1DForOutWhenUnconnected=off
  nlp.status : Outport  Port=6  VectorParamsAs1DForOutWhenUnconnected=off
  nlp.solvetime : Outport  Port=7  VectorParamsAs1DForOutWhenUnconnected=off
  solverid : Outport  Port=8  VectorParamsAs1DForOutWhenUnconnected=off
  X0 : Outport  Port=9  VectorParamsAs1DForOutWhenUnconnected=off
  MV0 : Outport  Port=10  VectorParamsAs1DForOutWhenUnconnected=off
  wires:
  NLMPC/10(MV0) -> MV0/1
  NLMPC/9(X0) -> X0/1
  ref/1 -> NLMPC/2(ref)
  Reshape1/1 -> NLMPC/3(lastMV)
  lastMV/1 -> Reshape1/1
  x/1 -> Reshape/1
  xinit/1 -> NLMPC/20("X0 ")
  mvinit/1 -> NLMPC/19("MV0 ")
  rhoeps/1 -> NLMPC/17(ECRWeight)
  duwt/1 -> NLMPC/16(MVRateWeights)
  uwt/1 -> NLMPC/15(MVWeights)
  ywt/1 -> NLMPC/14(OutputWeights)
  xmax/1 -> NLMPC/13(StateMax)
  xmin/1 -> NLMPC/12(StateMin)
  dumax/1 -> NLMPC/11(MVRateMax)
  dumin/1 -> NLMPC/10(MVRateMin)
  ymax/1 -> NLMPC/9(OutputMax)
  ymin/1 -> NLMPC/8(OutputMin)
  umax/1 -> NLMPC/7(MVMax)
  umin/1 -> NLMPC/6(MVMin)
  mv.target/1 -> NLMPC/5(MVTarget)
  md/1 -> NLMPC/4(md)
  Reshape/1 -> NLMPC/1(x)
  NLMPC/1(mv) -> mv/1
  NLMPC/6(nlpstatus) -> nlp.status/1
  NLMPC/5(yseq) -> y.seq/1
  NLMPC/4(xseq) -> x.seq/1
  NLMPC/3(mvseq) -> mv.seq/1
  NLMPC/2(cost) -> cost/1
  parameters/1 -> Reshape2/1
  Reshape2/1 -> NLMPC/18(Parameter)
  NLMPC/7(nlpsolvetime) -> nlp.solvetime/1
  NLMPC/8(solverid) -> solverid/1

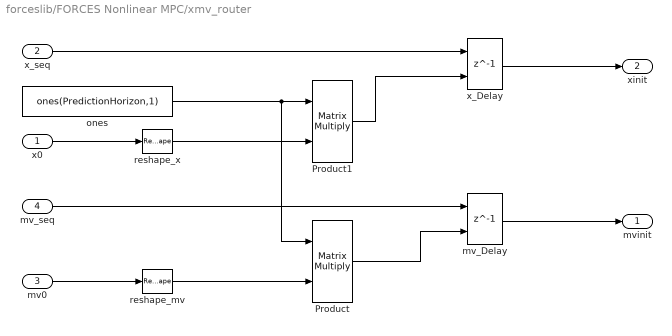
== system forceslib/FORCES Nonlinear MPC/xmv_router ==
  x0 : Inport
  x_seq : Inport  Port=2
  mv0 : Inport  Port=3
  mv_seq : Inport  Port=4
  Product : Product  Multiplication=Matrix(*)
  Product1 : Product  Multiplication=Matrix(*)
  mv_Delay : Delay  DelayLength=1  InitialConditionSource=Input port  SampleTime=Ts
      settings: InputPortMap=u0,p4
  ones : Constant  Value=ones(PredictionHorizon,1)  VectorParams1D=off
  reshape_mv : Reshape  OutputDimensionality=Row vector (2-D)
  reshape_x : Reshape  OutputDimensionality=Row vector (2-D)
  x_Delay : Delay  DelayLength=1  InitialConditionSource=Input port  SampleTime=Ts
      settings: InputPortMap=u0,p4
  mvinit : Outport  VectorParamsAs1DForOutWhenUnconnected=off
  xinit : Outport  Port=2  VectorParamsAs1DForOutWhenUnconnected=off
  wires:
  mv_Delay/1 -> mvinit/1
  x_Delay/1 -> xinit/1
  x_seq/1 -> x_Delay/1
  mv_seq/1 -> mv_Delay/1
  Product/1 -> mv_Delay/2
  Product1/1 -> x_Delay/2
  ones/1 -> Product/1, Product1/1
  reshape_x/1 -> Product1/2
  x0/1 -> reshape_x/1
  mv0/1 -> reshape_mv/1
  reshape_mv/1 -> Product/2

== matlab function forceslib/FORCES LTV MPC (Sparse QP)/MPC/Optimizer ==
  settings: updateMethod=DISCRETE  sampleTime=MPCstruct.Ts
  data: xkkm1 input double; lastmv input; xkkp1 output; moorx input; mv output; yref input; md input; extmv input; umin input; umax input; dumin input; dumax input; ymin input; ymax input; ywt input; uwt input; duwt input; ecrwt input; uref input; A input; B input; C input; D input; U input; Y input; X input; DX input; Pkk input; MPCstruct parameter; cost output; mvseq output; xseq output; yseq output; exitflag output; solvetime output; solverid output; xkk output; Pkk output
function [xkkp1,mv,cost,mvseq,xseq,yseq,exitflag,solvetime,solverid,xkk,Pkk] = fcn(xkkm1,lastmv,moorx,yref,md,extmv,umin,umax,dumin,dumax,ymin,ymax,ywt,uwt,duwt,ecrwt,uref,A,B,C,D,U,Y,X,DX,Pkk,MPCstruct)
    % Pre-allocate all the MEX block outputs for the simulation mode %#ok<*PREALL>
    [xkkp1,mv,cost,mvseq,xseq,yseq,exitflag,solvetime,solverid,xkk,Pkk] = mpcSparseSimulinkBlock(xkkm1,lastmv,moorx,yref,md,extmv,umin,umax,dumin,dumax,ymin,ymax,ywt,uwt,duwt,ecrwt,uref,A,B,C,D,U,Y,X,DX,Pkk,MPCstruct,MPCstruct.IsDummy,2);
end

== matlab function forceslib/FORCES Nonlinear MPC/MPC/NLMPC ==
  settings: updateMethod=DISCRETE  sampleTime=blkData.Ts
  data: x input; mv output; ref input; lastMV input; md input; MVTarget input; MVMin input; MVMax input; OutputMin input; OutputMax input; MVRateMin input; MVRateMax input; StateMin input; StateMax input; OutputWeights input; MVWeights input; MVRateWeights input; ECRWeight input; cost output size=[1,1]; mvseq output size=[blkData.p+1 blkData.nmv]; xseq output size=[blkData.p+1 blkData.nx]; yseq output size=[blkData.p+1 blkData.ny]; nlpstatus output size=[1,1]; nlpsolvetime output; solverid output; Parameter input; MV0 input size=[blkData.p blkData.nmv]; X0 input size=[blkData.p blkData.nx]; blkData parameter; X0 output; MV0 output
function [mv, cost, mvseq, xseq, yseq, nlpstatus, nlpsolvetime, solverid, X0, MV0] = fcn(x, ref, lastMV, md, MVTarget, ...
    MVMin, MVMax, OutputMin, OutputMax, MVRateMin, MVRateMax, StateMin, StateMax, ...
    OutputWeights, MVWeights, MVRateWeights, ECRWeight, Parameter, MV0, X0, blkData)
    
    % Calls NLP solver for Nonlinear MPC block
    [mv, cost, mvseq, xseq, yseq, nlpstatus, nlpsolvetime, solverid, X0, MV0] = nlmpcSimulinkBlock(x, ref, lastMV, md, MVTarget, ...
        MVMin, MVMax, OutputMin, OutputMax, MVRateMin, MVRateMax, StateMin, StateMax, ...
        OutputWeights, MVWeights, MVRateWeights, ECRWeight, Parameter, MV0, X0, blkData);
end

== matlab function forceslib/FORCES MPC (Sparse QP)/MPC/Optimizer ==
  settings: updateMethod=DISCRETE  sampleTime=MPCstruct.Ts
  data: xkkm1 input double; lastmv input; xkkp1 output; moorx input; mv output; yref input; md input; extmv input; umin input; umax input; dumin input; dumax input; ymin input; ymax input; ywt input; uwt input; duwt input; ecrwt input; uref input; Pkk input; MPCstruct parameter; cost output; mvseq output; xseq output; yseq output; exitflag output; solvetime output; solverid output; xkk output
function [xkkp1,mv,cost,mvseq,xseq,yseq,exitflag,solvetime,solverid,xkk] = fcn(xkkm1,lastmv,moorx,yref,md,extmv,umin,umax,dumin,dumax,ymin,ymax,ywt,uwt,duwt,ecrwt,uref,Pkk,MPCstruct)
    % Pre-allocate all the MEX block outputs for the simulation mode %#ok<*PREALL>
    [xkkp1,mv,cost,mvseq,xseq,yseq,exitflag,solvetime,solverid,xkk,~] = mpcSparseSimulinkBlock(xkkm1,lastmv,moorx,yref,md,extmv,umin,umax,dumin,dumax,ymin,ymax,ywt,uwt,duwt,ecrwt,uref,0,0,0,0,0,0,0,0,Pkk,MPCstruct,MPCstruct.IsDummy,0);
end

== matlab function forceslib/FORCES ADAPTIVE MPC (Sparse QP)/MPC/Optimizer ==
  settings: updateMethod=DISCRETE  sampleTime=MPCstruct.Ts
  data: xkkm1 input double; lastmv input; xkkp1 output; moorx input; mv output; yref input; md input; extmv input; umin input; umax input; dumin input; dumax input; ymin input; ymax input; ywt input; uwt input; duwt input; ecrwt input; uref input; A input; B input; C input; D input; U input; Y input; X input; DX input; Pkk input; MPCstruct parameter; cost output; mvseq output; xseq output; yseq output; exitflag output; solvetime output; solverid output; xkk output; Pkk output
function [xkkp1,mv,cost,mvseq,xseq,yseq,exitflag,solvetime,solverid,xkk,Pkk] = fcn(xkkm1,lastmv,moorx,yref,md,extmv,umin,umax,dumin,dumax,ymin,ymax,ywt,uwt,duwt,ecrwt,uref,A,B,C,D,U,Y,X,DX,Pkk,MPCstruct)
    % Pre-allocate all the MEX block outputs for the simulation mode %#ok<*PREALL>
    [xkkp1,mv,cost,mvseq,xseq,yseq,exitflag,solvetime,solverid,xkk,Pkk] = mpcSparseSimulinkBlock(xkkm1,lastmv,moorx,yref,md,extmv,umin,umax,dumin,dumax,ymin,ymax,ywt,uwt,duwt,ecrwt,uref,A,B,C,D,U,Y,X,DX,Pkk,MPCstruct,MPCstruct.IsDummy,1);
end
